simulink subsystem "rss_ElecAgElecSpdMgAndPredElecSpdCmpt"  (R2023a)
settings: Solver=VariableStepAuto  StartTime=0.0  StopTime=10.0  RelTol=1e-3
undefined symbols (not defined in the file): bit, Cdbl_facOpnLpClsLpAgRiseRateMaxVal, Cdbl_fEstAgDvtCompFrqMaxVal, Cdbl_nElecAgSpdMaxVal, Cdbl_nElecAgSpdPeakVal, Cdbl_phiEstElecAgDvtMaxVal, Cdbl_tiMedTaskSmpTi, ENM_AG_POS_EVAL_MODE, ENM_MOTO_STATUS, Gs16_facOpnLpClsLpAgRiseRate_C, Gs16_nSenlTrnsElecSpd_C, Gu16_ctSenlTrnsElecAgConfCnt_C, Gu16_ctSenlTrnsElecAgRcvyCnt_C, Gu16_phiMaxSenlTrnsElecAg_C
libraries: simulink x7, lib_conversion x6, lib_configurable_parameter x2, lib_discrete_time_integrator x1, lib_debounce x1, lib_iir_filter x1
settings Model: Creator=xiaoqiang.yuan  LastModifiedBy=xiaoqiang.yuan

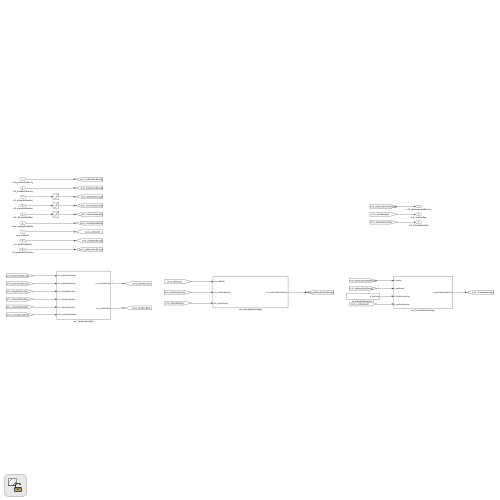
[thumbnail: Simulink's stored preview of the top-level diagram]
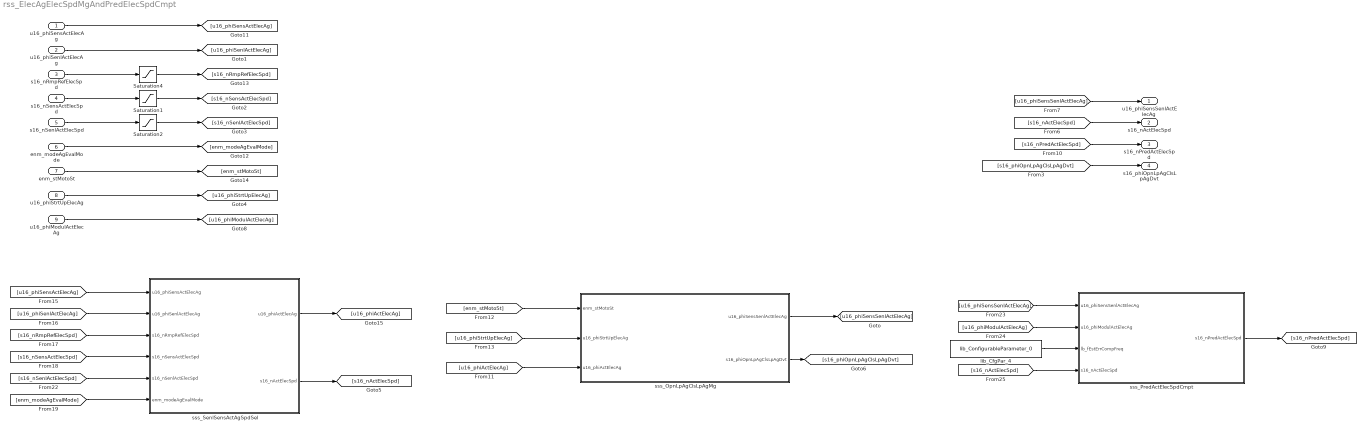
== system rss_ElecAgElecSpdMgAndPredElecSpdCmpt ==
  u16_phiSensActElecAg : Inport  OutDataTypeStr=dt_RadAng_u16r15b0
  u16_phiSenlActElecAg : Inport  Port=2  OutDataTypeStr=dt_RadAng_u16r15b0
  s16_nRmpRefElecSpd : Inport  Port=3  OutDataTypeStr=dt_Standardize_s16p15b0
  s16_nSensActElecSpd : Inport  Port=4  OutDataTypeStr=dt_Standardize_s16p15b0
  s16_nSenlActElecSpd : Inport  Port=5  OutDataTypeStr=dt_Standardize_s16p15b0
  enm_modeAgEvalMode : Inport  Port=6  OutDataTypeStr=Enum: ENM_AG_POS_EVAL_MODE
  enm_stMotoSt : Inport  Port=7  OutDataTypeStr=Enum: ENM_MOTO_STATUS
  u16_phiStrtUpElecAg : Inport  Port=8  OutDataTypeStr=dt_RadAng_u16r15b0
  u16_phiModulActElecAg : Inport  Port=9  OutDataTypeStr=dt_RadAng_u16r15b0
  Saturation1 : Saturate  UpperLimit=Cdbl_nElecAgSpdMaxVal  LowerLimit=-Cdbl_nElecAgSpdMaxVal
  Saturation2 : Saturate  UpperLimit=Cdbl_nElecAgSpdMaxVal  LowerLimit=-Cdbl_nElecAgSpdMaxVal
  Saturation4 : Saturate  UpperLimit=Cdbl_nElecAgSpdMaxVal  LowerLimit=-Cdbl_nElecAgSpdMaxVal
  lib_CfgPar_4 : lib_configurable_parameter/lib_ConfigurableParameter_0  lb_parCnfgPar=Gu16_fEstAgDvtCompFrq_C  lb_parDataType=Inherit: Inherit from 'Constant value'  lb_parUpLim=Cdbl_fEstAgDvtCompFrqMaxVal  lb_parLowLim=Cdbl_fEstAgDvtCompFrqMinVal
  sss_OpnLpAgClsLpAgMg : Subsystem
  sss_PredActElecSpdCmpt : Subsystem
  sss_SenlSensActAgSpdSel : Subsystem
  u16_phiSensSenlActElecAg : Outport  OutDataTypeStr=dt_RadAng_u16r15b0
  s16_nActElecSpd : Outport  Port=2  OutDataTypeStr=dt_Standardize_s16p15b0
  s16_nPredActElecSpd : Outport  Port=3  OutDataTypeStr=dt_Standardize_s16p15b0  PortDimensions=1  VectorParamsAs1DForOutWhenUnconnected=off
  s16_phiOpnLpAgClsLpAgDvt : Outport  Port=4
  wires:
  u16_phiSensActElecAg/1 -> [u16_phiSensActElecAg]
  u16_phiSenlActElecAg/1 -> [u16_phiSenlActElecAg]
  s16_nRmpRefElecSpd/1 -> Saturation4/1
  Saturation4/1 -> [s16_nRmpRefElecSpd]
  Saturation1/1 -> [s16_nSensActElecSpd]
  s16_nSensActElecSpd/1 -> Saturation1/1
  s16_nSenlActElecSpd/1 -> Saturation2/1
  Saturation2/1 -> [s16_nSenlActElecSpd]
  enm_modeAgEvalMode/1 -> [enm_modeAgEvalMode]
  enm_stMotoSt/1 -> [enm_stMotoSt]
  u16_phiStrtUpElecAg/1 -> [u16_phiStrtUpElecAg]
  u16_phiModulActElecAg/1 -> [u16_phiModulActElecAg]
  [s16_nActElecSpd] -> s16_nActElecSpd/1
  [u16_phiSensSenlActElecAg] -> u16_phiSensSenlActElecAg/1
  [s16_nPredActElecSpd] -> s16_nPredActElecSpd/1
  [enm_modeAgEvalMode] -> sss_SenlSensActAgSpdSel/6(enm_modeAgEvalMode)
  [u16_phiSenlActElecAg] -> sss_SenlSensActAgSpdSel/2(u16_phiSenlActElecAg)
  [s16_nRmpRefElecSpd] -> sss_SenlSensActAgSpdSel/3(s16_nRmpRefElecSpd)
  [enm_stMotoSt] -> sss_OpnLpAgClsLpAgMg/1(enm_stMotoSt)
  [u16_phiStrtUpElecAg] -> sss_OpnLpAgClsLpAgMg/2(u16_phiStrtUpElecAg)
  [s16_nSensActElecSpd] -> sss_SenlSensActAgSpdSel/4(s16_nSensActElecSpd)
  [s16_nSenlActElecSpd] -> sss_SenlSensActAgSpdSel/5(s16_nSenlActElecSpd)
  [s16_nActElecSpd] -> sss_PredActElecSpdCmpt/4(s16_nActElecSpd)
  [u16_phiModulActElecAg] -> sss_PredActElecSpdCmpt/2(u16_phiModulActElecAg)
  [u16_phiSensSenlActElecAg] -> sss_PredActElecSpdCmpt/1(u16_phiSensSenlActElecAg)
  [u16_phiSensActElecAg] -> sss_SenlSensActAgSpdSel/1(u16_phiSensActElecAg)
  [u16_phiActElecAg] -> sss_OpnLpAgClsLpAgMg/3(u16_phiActElecAg)
  lib_CfgPar_4/1 -> sss_PredActElecSpdCmpt/3(lb_fEstErrCompFreq)
  sss_PredActElecSpdCmpt/1(s16_nPredActElecSpd) -> [s16_nPredActElecSpd]
  sss_SenlSensActAgSpdSel/1(u16_phiActElecAg) -> [u16_phiActElecAg]
  sss_SenlSensActAgSpdSel/2(s16_nActElecSpd) -> [s16_nActElecSpd]
  sss_OpnLpAgClsLpAgMg/1(u16_phiSensSenlActElecAg) -> [u16_phiSensSenlActElecAg]
  sss_OpnLpAgClsLpAgMg/2(s16_phiOpnLpAgClsLpAgDvt) -> [s16_phiOpnLpAgClsLpAgDvt]
  [s16_phiOpnLpAgClsLpAgDvt] -> s16_phiOpnLpAgClsLpAgDvt/1

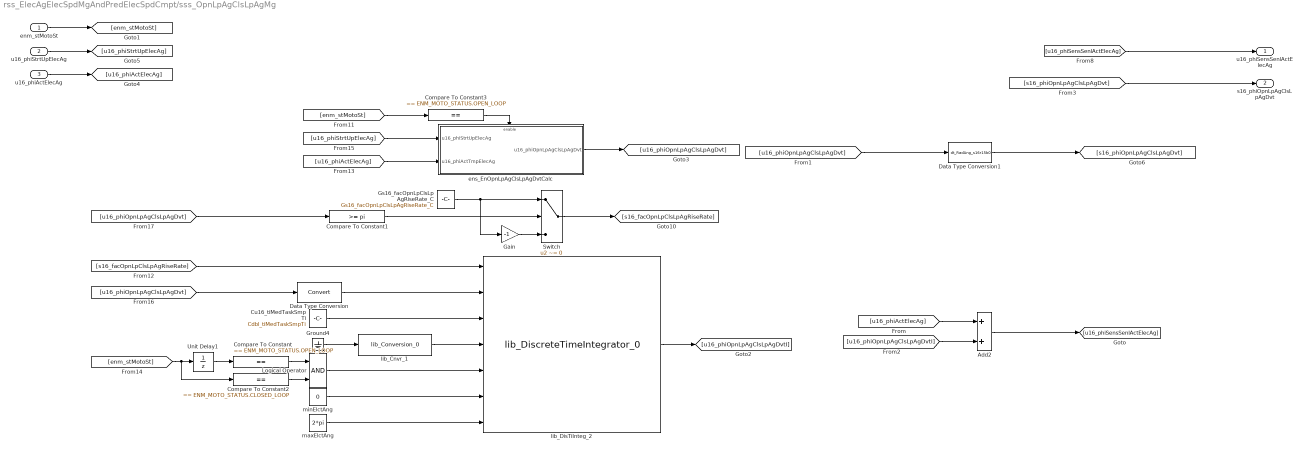
== system rss_ElecAgElecSpdMgAndPredElecSpdCmpt/sss_OpnLpAgClsLpAgMg ==
  enm_stMotoSt : Inport
  u16_phiStrtUpElecAg : Inport  Port=2
  u16_phiActElecAg : Inport  Port=3
  Add2 : Sum  InitFcn=|  OutDataTypeStr=Inherit: Same as first input
      | Simulink.suppressDiagnostic(gcb,...
      | 'SimulinkFixedPoint:util:Overflowoccurred');
  Compare To Constant : simulink/Logic and Bit Operations/Compare To Constant  relop===  const=ENM_MOTO_STATUS.OPEN_LOOP  OutDataTypeStr=boolean
  Compare To Constant1 : simulink/Logic and Bit Operations/Compare To Constant  relop=>=  const=pi  OutDataTypeStr=boolean
  Compare To Constant2 : simulink/Logic and Bit Operations/Compare To Constant  relop===  const=ENM_MOTO_STATUS.CLOSED_LOOP  OutDataTypeStr=boolean
  Compare To Constant3 : simulink/Logic and Bit Operations/Compare To Constant  relop===  const=ENM_MOTO_STATUS.OPEN_LOOP  OutDataTypeStr=boolean
  Cu16_tiMedTaskSmpTi : Constant  Value=Cdbl_tiMedTaskSmpTi
  Data Type Conversion : DataTypeConversion  SaturateOnIntegerOverflow=off  RndMeth=Floor
  Data Type Conversion1 : DataTypeConversion  OutDataTypeStr=dt_RadAng_s16r15b0  SaturateOnIntegerOverflow=off  RndMeth=Floor
  Gain : Gain  Gain=-1  OutDataTypeStr=Inherit: Same as input
  Ground4 : Ground
  Gs16_facOpnLpClsLpAgRiseRate_C : Constant  Value=Gs16_facOpnLpClsLpAgRiseRate_C  OutDataTypeStr=fixdt(1,16,2^-2,0)
  Logical Operator : Logic  AllPortsSameDT=off  OutDataTypeStr=boolean
  Switch : Switch  Criteria=u2 ~= 0  SaturateOnIntegerOverflow=off  InputSameDT=off  OutDataTypeStr=Inherit: Same as first input
  Unit Delay1 : UnitDelay  InitialCondition=ENM_MOTO_STATUS.OFF  SampleTime=-1  HasFrameUpgradeWarning=on
  ens_EnOpnLpAgClsLpAgDvtCalc : Subsystem
  lib_Cnvr_1 : lib_conversion/lib_Conversion_0  lb_parDataType=uint8  lb_parOutpMaxVal=[]  lb_parOutpMinVal=[]  lb_parSatFlag=off
  lib_DisTiInteg_2 : lib_discrete_time_integrator/lib_DiscreteTimeIntegrator_0  lb_parMaxInpVal=Cdbl_facOpnLpClsLpAgRiseRateMaxVal  lb_parMinInpVal=-Cdbl_facOpnLpClsLpAgRiseRateMaxVal  lb_parMaxSampTime=double(Cdbl_tiMedTaskSmpTi)  lb_parMaxIntgGain=0  lb_parAccmDataTypeMode=Same of output  lb_parOutpDataType=dt_RadAngErr_s16r13b0  lb_parIntgScopMode=Generic signal  lb_parSatFlag=on
  maxElctAng : Constant  Value=2*pi  OutDataTypeStr=Inherit: Inherit via back propagation
  minElctAng : Constant  Value=0  OutDataTypeStr=Inherit: Inherit via back propagation
  u16_phiSensSenlActElecAg : Outport
  s16_phiOpnLpAgClsLpAgDvt : Outport  Port=2
  wires:
  [s16_phiOpnLpAgClsLpAgDvt] -> s16_phiOpnLpAgClsLpAgDvt/1
  Data Type Conversion1/1 -> [s16_phiOpnLpAgClsLpAgDvt]
  [u16_phiOpnLpAgClsLpAgDvt] -> Data Type Conversion1/1
  Ground4/1 -> lib_Cnvr_1/1
  Gain/1 -> Switch/3
  Gs16_facOpnLpClsLpAgRiseRate_C/1 -> Gain/1, Switch/1
  Add2/1 -> [u16_phiSensSenlActElecAg]
  Compare To Constant3/1 -> ens_EnOpnLpAgClsLpAgDvtCalc/Enable
  [u16_phiOpnLpAgClsLpAgDvtI] -> Add2/2
  [u16_phiActElecAg] -> Add2/1
  [u16_phiSensSenlActElecAg] -> u16_phiSensSenlActElecAg/1
  u16_phiActElecAg/1 -> [u16_phiActElecAg]
  u16_phiStrtUpElecAg/1 -> [u16_phiStrtUpElecAg]
  enm_stMotoSt/1 -> [enm_stMotoSt]
  ens_EnOpnLpAgClsLpAgDvtCalc/1(u16_phiOpnLpAgClsLpAgDvt) -> [u16_phiOpnLpAgClsLpAgDvt]
  Switch/1 -> [s16_facOpnLpClsLpAgRiseRate]
  [u16_phiOpnLpAgClsLpAgDvt] -> Data Type Conversion/1
  [enm_stMotoSt] -> Compare To Constant3/1
  lib_DisTiInteg_2/1 -> [u16_phiOpnLpAgClsLpAgDvtI]
  Unit Delay1/1 -> Compare To Constant/1
  [u16_phiOpnLpAgClsLpAgDvt] -> Compare To Constant1/1
  [u16_phiStrtUpElecAg] -> ens_EnOpnLpAgClsLpAgDvtCalc/1(u16_phiStrtUpElecAg)
  maxElctAng/1 -> lib_DisTiInteg_2/7
  [enm_stMotoSt] -> Compare To Constant2/1, Unit Delay1/1
  [u16_phiActElecAg] -> ens_EnOpnLpAgClsLpAgDvtCalc/2(u16_phiActTmpElecAg)
  Logical Operator/1 -> lib_DisTiInteg_2/5
  Compare To Constant1/1 -> Switch/2
  Compare To Constant/1 -> Logical Operator/1
  minElctAng/1 -> lib_DisTiInteg_2/6
  [s16_facOpnLpClsLpAgRiseRate] -> lib_DisTiInteg_2/1
  Cu16_tiMedTaskSmpTi/1 -> lib_DisTiInteg_2/3
  Compare To Constant2/1 -> Logical Operator/2
  lib_Cnvr_1/1 -> lib_DisTiInteg_2/4
  Data Type Conversion/1 -> lib_DisTiInteg_2/2

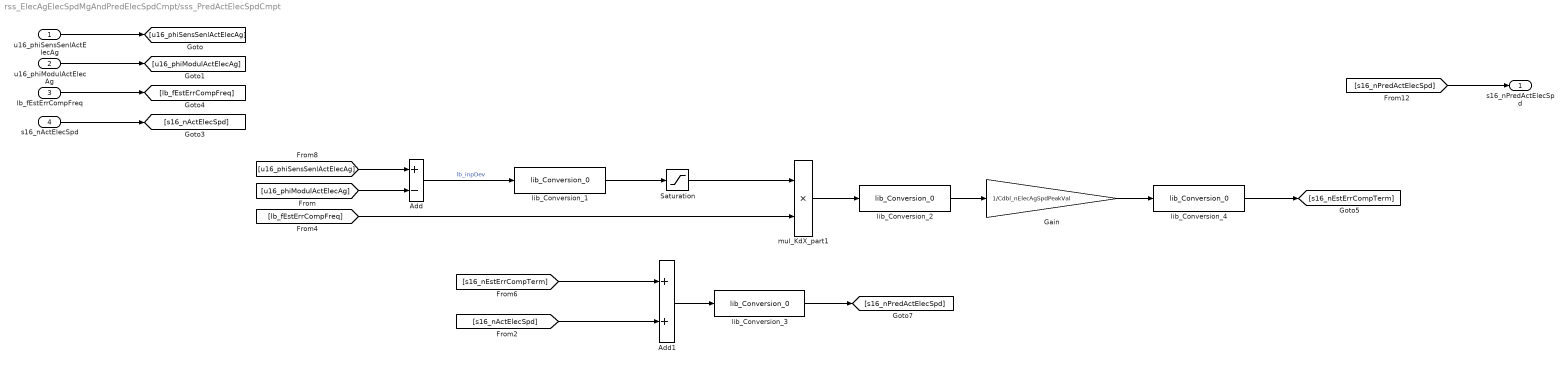
== system rss_ElecAgElecSpdMgAndPredElecSpdCmpt/sss_PredActElecSpdCmpt ==
  u16_phiSensSenlActElecAg : Inport  PortDimensions=1
  u16_phiModulActElecAg : Inport  Port=2  PortDimensions=1
  lb_fEstErrCompFreq : Inport  Port=3
  s16_nActElecSpd : Inport  Port=4
  Add : Sum  Inputs=+-  OutDataTypeStr=Inherit: Inherit via back propagation  RndMeth=Simplest
  Add1 : Sum  OutDataTypeStr=Inherit: Inherit via back propagation  RndMeth=Simplest
  Gain : Gain  Gain=1/Cdbl_nElecAgSpdPeakVal  OutDataTypeStr=Inherit: Inherit via back propagation
  Saturation : Saturate  UpperLimit=Cdbl_phiEstElecAgDvtMaxVal  LowerLimit=-Cdbl_phiEstElecAgDvtMaxVal
  lib_Conversion_1 : lib_conversion/lib_Conversion_0  lb_parDataType=fixdt(1,16,pi*2^-15,0)  lb_parOutpMaxVal=[]  lb_parOutpMinVal=[]  lb_parSatFlag=off
  lib_Conversion_2 : lib_conversion/lib_Conversion_0  lb_parDataType=fixdt(1,16)  lb_parOutpMaxVal=Cdbl_phiEstElecAgDvtMaxVal*Cdbl_fEstAgDvtCompFrqMaxVal  lb_parOutpMinVal=[]  lb_parSatFlag=off
  lib_Conversion_3 : lib_conversion/lib_Conversion_0  lb_parDataType=dt_Standardize_s16p15b0  lb_parOutpMaxVal=[]  lb_parOutpMinVal=[]  lb_parSatFlag=off
  lib_Conversion_4 : lib_conversion/lib_Conversion_0  lb_parDataType=dt_Standardize_s16p15b0  lb_parOutpMaxVal=[]  lb_parOutpMinVal=[]  lb_parSatFlag=off
  mul_KdX_part1 : Product  OutDataTypeStr=Inherit: Inherit via back propagation  RndMeth=Simplest
  s16_nPredActElecSpd : Outport  PortDimensions=1  VectorParamsAs1DForOutWhenUnconnected=off
  wires:
  lib_Conversion_1/1 -> Saturation/1
  [s16_nActElecSpd] -> Add1/2
  mul_KdX_part1/1 -> lib_Conversion_2/1
  [u16_phiSensSenlActElecAg] -> Add/1
  [u16_phiModulActElecAg] -> Add/2
  [s16_nEstErrCompTerm] -> Add1/1
  [s16_nPredActElecSpd] -> s16_nPredActElecSpd/1
  u16_phiSensSenlActElecAg/1 -> [u16_phiSensSenlActElecAg]
  lib_Conversion_2/1 -> Gain/1
  [lb_fEstErrCompFreq] -> mul_KdX_part1/2
  s16_nActElecSpd/1 -> [s16_nActElecSpd]
  u16_phiModulActElecAg/1 -> [u16_phiModulActElecAg]
  Add/1 -> lib_Conversion_1/1  "lb_inpDev"
  Saturation/1 -> mul_KdX_part1/1
  lb_fEstErrCompFreq/1 -> [lb_fEstErrCompFreq]
  Add1/1 -> lib_Conversion_3/1
  lib_Conversion_3/1 -> [s16_nPredActElecSpd]
  Gain/1 -> lib_Conversion_4/1
  lib_Conversion_4/1 -> [s16_nEstErrCompTerm]

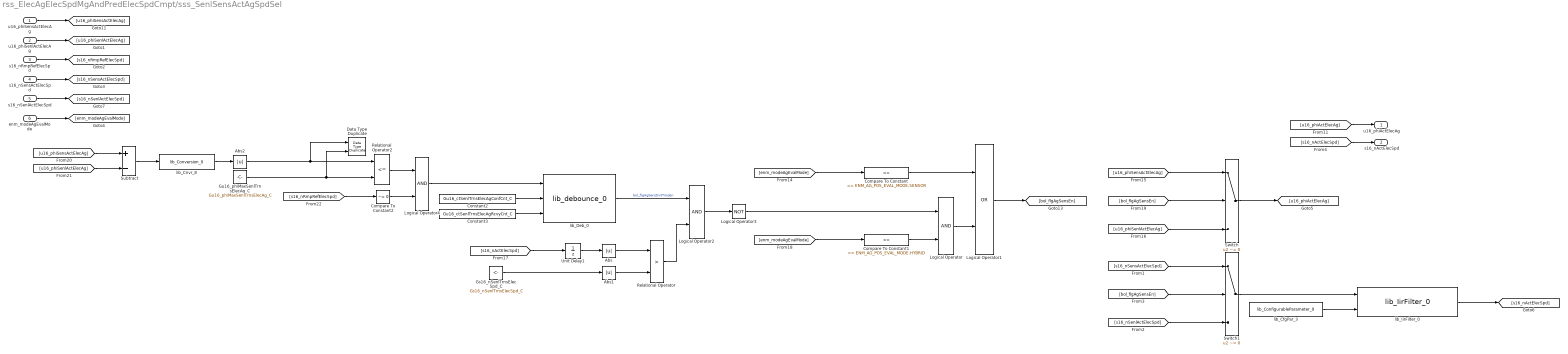
== system rss_ElecAgElecSpdMgAndPredElecSpdCmpt/sss_SenlSensActAgSpdSel ==
  u16_phiSensActElecAg : Inport
  u16_phiSenlActElecAg : Inport  Port=2
  s16_nRmpRefElecSpd : Inport  Port=3
  s16_nSensActElecSpd : Inport  Port=4
  s16_nSenlActElecSpd : Inport  Port=5
  enm_modeAgEvalMode : Inport  Port=6
  Abs : Abs  SaturateOnIntegerOverflow=off
  Abs1 : Abs  SaturateOnIntegerOverflow=off
  Abs2 : Abs  OutDataTypeStr=Inherit: Inherit via back propagation  SaturateOnIntegerOverflow=off
  Compare To Constant : simulink/Logic and Bit Operations/Compare To Constant  relop===  const=ENM_AG_POS_EVAL_MODE.SENSOR  OutDataTypeStr=boolean
  Compare To Constant1 : simulink/Logic and Bit Operations/Compare To Constant  relop===  const=ENM_AG_POS_EVAL_MODE.HYBRID  OutDataTypeStr=boolean
  Compare To Constant2 : simulink/Logic and Bit Operations/Compare To Constant  relop=~=  const=0  OutDataTypeStr=boolean
  Constant2 : Constant  Value=Gu16_ctSenlTrnsElecAgConfCnt_C
  Constant3 : Constant  Value=Gu16_ctSenlTrnsElecAgRcvyCnt_C
  Data Type Duplicate : DataTypeDuplicate
  Gs16_nSenlTrnsElecSpd_C : Constant  Value=Gs16_nSenlTrnsElecSpd_C
  Gu16_phiMaxSenlTrnsElecAg_C : Constant  Value=Gu16_phiMaxSenlTrnsElecAg_C
  Logical Operator : Logic  AllPortsSameDT=off  OutDataTypeStr=boolean
  Logical Operator1 : Logic  Operator=OR  AllPortsSameDT=off  OutDataTypeStr=boolean
  Logical Operator2 : Logic  AllPortsSameDT=off  OutDataTypeStr=boolean
  Logical Operator3 : Logic  Operator=NOT  AllPortsSameDT=off  OutDataTypeStr=boolean
  Logical Operator4 : Logic  AllPortsSameDT=off  OutDataTypeStr=boolean
  Relational Operator : RelationalOperator  Operator=>  OutDataTypeStr=boolean  RndMeth=Simplest  InputSameDT=off
  Relational Operator2 : RelationalOperator  Operator=<=  OutDataTypeStr=boolean  RndMeth=Simplest  InputSameDT=off
  Subtract : Sum  Inputs=+-  OutDataTypeStr=Inherit: Inherit via back propagation
  Switch : Switch  Criteria=u2 ~= 0  SaturateOnIntegerOverflow=off  InputSameDT=off
  Switch1 : Switch  Criteria=u2 ~= 0  SaturateOnIntegerOverflow=off  InputSameDT=off
  Unit Delay1 : UnitDelay  SampleTime=-1  HasFrameUpgradeWarning=on
  lib_CfgPar_3 : lib_configurable_parameter/lib_ConfigurableParameter_0  lb_parCnfgPar=Gu16_facSpdFltCoeff_C  lb_parDataType=Inherit: Inherit from 'Constant value'  lb_parUpLim=Cdbl_facSpdFltCoeffMaxVal  lb_parLowLim=Cdbl_facSpdFltCoeffMinVal
  lib_Cnvr_8 : lib_conversion/lib_Conversion_0  lb_parDataType=fixdt(1,16,pi*2^-15,0)  lb_parOutpMaxVal=[]  lb_parOutpMinVal=[]  lb_parSatFlag=off
  lib_Deb_0 : lib_debounce/lib_debounce_0
  lib_IirFilter_0 : lib_iir_filter/lib_IirFilter_0  lb_parMaxInpVal=Cdbl_nElecAgSpdMaxVal  lb_parFltrCoefMaxVal=Cdbl_facSpdFltCoeffMaxVal  lb_parBitNumMode=16-bit  lb_parOutpDataType=dt_Standardize_s16p15b0  lb_parFiltTypeMode=Low-pass
  u16_phiActElecAg : Outport
  s16_nActElecSpd : Outport  Port=2
  wires:
  Abs2/1 -> Relational Operator2/1, Data Type Duplicate/1
  lib_IirFilter_0/1 -> [s16_nActElecSpd]
  Switch1/1 -> lib_IirFilter_0/1
  lib_CfgPar_3/1 -> lib_IirFilter_0/2
  s16_nSenlActElecSpd/1 -> [s16_nSenlActElecSpd]
  Unit Delay1/1 -> Abs/1
  [s16_nActElecSpd] -> s16_nActElecSpd/1
  [bol_flgAgSensEn] -> Switch1/2
  [s16_nSensActElecSpd] -> Switch1/1
  [s16_nSenlActElecSpd] -> Switch1/3
  Abs/1 -> Relational Operator/1
  [u16_phiSenlActElecAg] -> Switch/3
  Switch/1 -> [u16_phiActElecAg]
  [u16_phiSensActElecAg] -> Switch/1
  [bol_flgAgSensEn] -> Switch/2
  [s16_nActElecSpd] -> Unit Delay1/1
  Gs16_nSenlTrnsElecSpd_C/1 -> Abs1/1
  [enm_modeAgEvalMode] -> Compare To Constant1/1
  [enm_modeAgEvalMode] -> Compare To Constant/1
  Constant3/1 -> lib_Deb_0/3
  Compare To Constant1/1 -> Logical Operator/2
  Constant2/1 -> lib_Deb_0/2
  Compare To Constant/1 -> Logical Operator1/1
  Abs1/1 -> Relational Operator/2
  Logical Operator4/1 -> lib_Deb_0/1
  [u16_phiSenlActElecAg] -> Subtract/2
  Gu16_phiMaxSenlTrnsElecAg_C/1 -> Relational Operator2/2, Data Type Duplicate/2
  [u16_phiSensActElecAg] -> Subtract/1
  lib_Deb_0/1 -> Logical Operator2/1  "bol_flgAgSensDvtTmpEn"
  lib_Cnvr_8/1 -> Abs2/1
  Relational Operator/1 -> Logical Operator2/2
  Logical Operator2/1 -> Logical Operator3/1
  Logical Operator3/1 -> Logical Operator/1
  Logical Operator1/1 -> [bol_flgAgSensEn]
  [s16_nRmpRefElecSpd] -> Compare To Constant2/1
  Subtract/1 -> lib_Cnvr_8/1
  Compare To Constant2/1 -> Logical Operator4/2
  Logical Operator/1 -> Logical Operator1/2
  Relational Operator2/1 -> Logical Operator4/1
  [u16_phiActElecAg] -> u16_phiActElecAg/1
  enm_modeAgEvalMode/1 -> [enm_modeAgEvalMode]
  s16_nSensActElecSpd/1 -> [s16_nSensActElecSpd]
  s16_nRmpRefElecSpd/1 -> [s16_nRmpRefElecSpd]
  u16_phiSenlActElecAg/1 -> [u16_phiSenlActElecAg]
  u16_phiSensActElecAg/1 -> [u16_phiSensActElecAg]

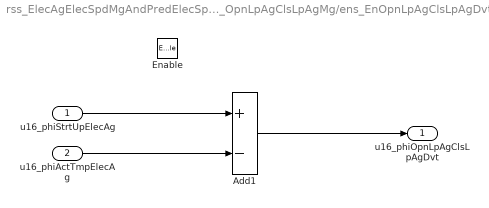
== system rss_ElecAgElecSpdMgAndPredElecSpdCmpt/sss_OpnLpAgClsLpAgMg/ens_EnOpnLpAgClsLpAgDvtCalc ==
  u16_phiStrtUpElecAg : Inport
  u16_phiActTmpElecAg : Inport  Port=2
  Enable : EnablePort
  Add1 : Sum  InitFcn=|  Inputs=+-  OutDataTypeStr=Inherit: Same as first input
      | Simulink.suppressDiagnostic(gcb,...
      | 'SimulinkFixedPoint:util:Overflowoccurred');
  u16_phiOpnLpAgClsLpAgDvt : Outport
  wires:
  Add1/1 -> u16_phiOpnLpAgClsLpAgDvt/1
  u16_phiStrtUpElecAg/1 -> Add1/1
  u16_phiActTmpElecAg/1 -> Add1/2
